simulink model "deployable"  (R2022a)
settings: Solver=VariableStepAuto  StartTime=0.0  StopTime=2  RelTol=1e-3
values from neighbouring files (symbols this model uses):
  mass_cart = 2    [Scuffscale_Values.m]
undefined symbols (not defined in the file or in its folder): KX
settings Model: Creator=josepfamador  LastModifiedBy=adrbe
settings DebuggingCC: UnconnectedInputMsg=warning  UnconnectedOutputMsg=warning  UnconnectedLineMsg=warning
settings RTWCC: DLArmComputeVersion=19.05

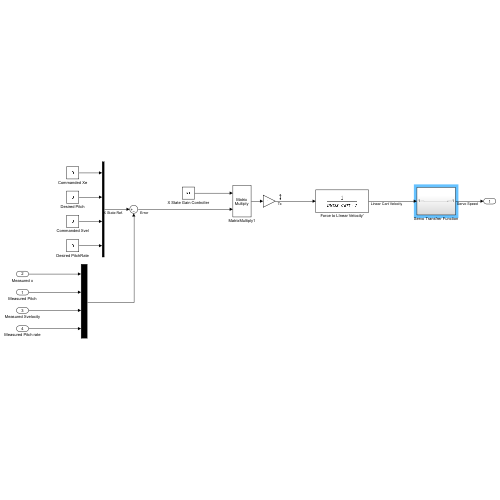
[thumbnail: Simulink's stored preview of the top-level diagram]
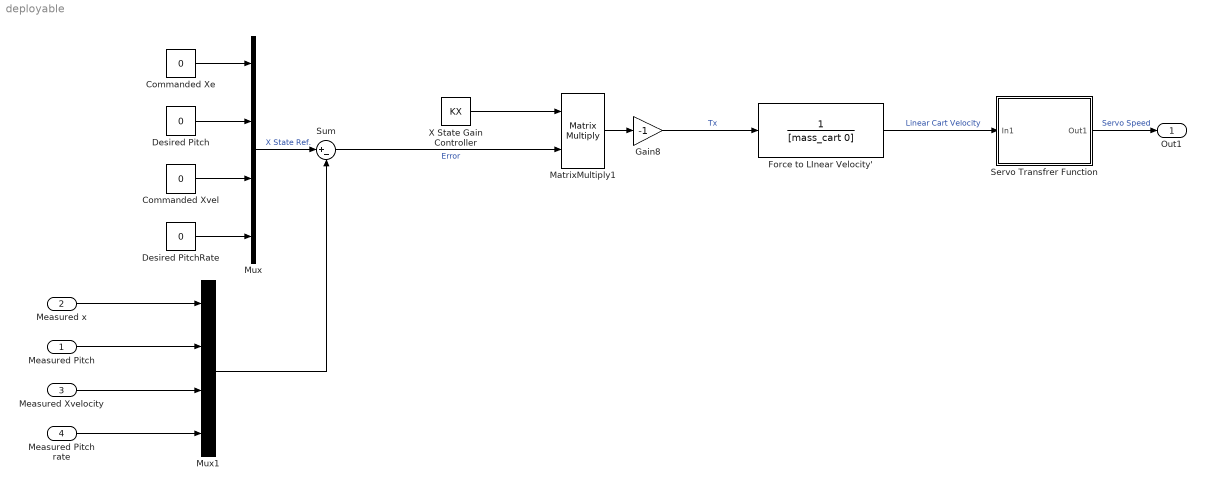
== system deployable ==
  Measured Pitch : Inport
  Measured x : Inport  Port=2
  Measured Xvelocity : Inport  Port=3
  Measured Pitch rate : Inport  Port=4
  Commanded Xe : Constant  Value=0
  Commanded Xvel : Constant  Value=0
  Desired Pitch : Constant  Value=0
  Desired PitchRate : Constant  Value=0
  Force to LInear Velocity' : TransferFcn  Denominator=[mass_cart 0]
  Gain8 : Gain  Gain=-1
  MatrixMultiply1 : Product  Multiplication=Matrix(*)
  Mux : Mux
  Mux1 : Mux
  Servo Transfrer Function : Subsystem
  Sum : Sum  Inputs=|+-
  X State Gain Controller : Constant  Value=KX  VectorParams1D=off
  Out1 : Outport
  wires:
  Sum/1 -> MatrixMultiply1/2  "Error"
  Commanded Xe/1 -> Mux/1
  Commanded Xvel/1 -> Mux/3
  Desired Pitch/1 -> Mux/2
  Mux/1 -> Sum/1  "X State Ref."
  Desired PitchRate/1 -> Mux/4
  X State Gain Controller/1 -> MatrixMultiply1/1
  MatrixMultiply1/1 -> Gain8/1
  Measured x/1 -> Mux1/1
  Measured Pitch/1 -> Mux1/2
  Measured Xvelocity/1 -> Mux1/3
  Measured Pitch rate/1 -> Mux1/4
  Mux1/1 -> Sum/2
  Gain8/1 -> Force to LInear Velocity'/1  "Tx"
  Force to LInear Velocity'/1 -> Servo Transfrer Function/1(In1)  "Linear Cart Velocity"
  Servo Transfrer Function/1(Out1) -> Out1/1  "Servo Speed"

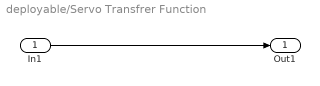
== system deployable/Servo Transfrer Function ==
  In1 : Inport
  Out1 : Outport
  wires:
  In1/1 -> Out1/1
